simulink model "demon_sim1"  (R2021b)
settings: Solver=VariableStepAuto  StartTime=0.0  StopTime=1.0  RelTol=1e-3
settings Model: Creator=Саня  LastModifiedBy=roman

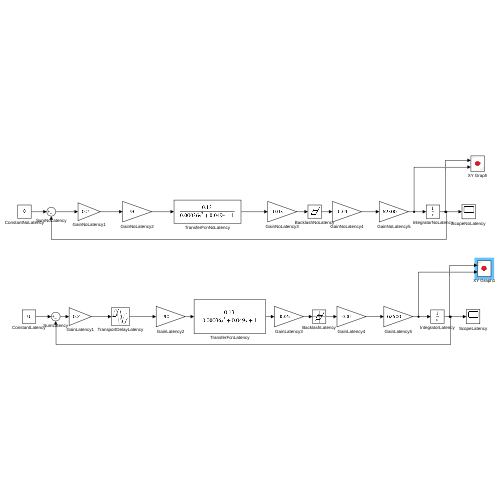
[thumbnail: Simulink's stored preview of the top-level diagram]
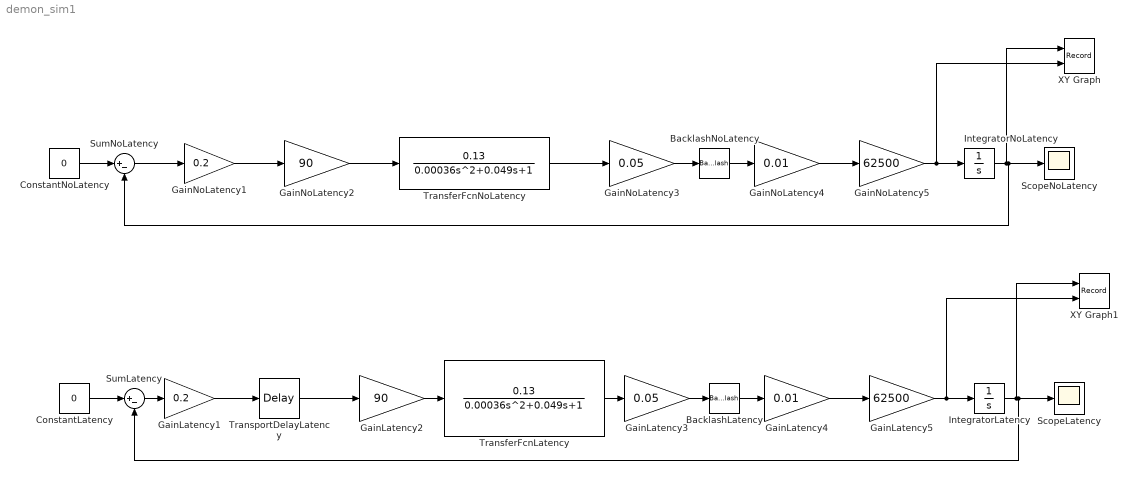
== system demon_sim1 ==
  BacklashLatency : Backlash  BacklashWidth=1e-6
  BacklashNoLatency : Backlash  BacklashWidth=1e-6
  ConstantLatency : Constant  Value=0
  ConstantNoLatency : Constant  Value=0
  GainLatency1 : Gain  Gain=0.2
  GainLatency2 : Gain  Gain=90
  GainLatency3 : Gain  Gain=0.05
  GainLatency4 : Gain  Gain=0.01
  GainLatency5 : Gain  Gain=62500
  GainNoLatency1 : Gain  Gain=0.2
  GainNoLatency2 : Gain  Gain=90  ParamDataTypeStr=double
  GainNoLatency3 : Gain  Gain=0.05
  GainNoLatency4 : Gain  Gain=0.01
  GainNoLatency5 : Gain  Gain=62500
  IntegratorLatency : Integrator  InitialCondition=13600
  IntegratorNoLatency : Integrator  InitialCondition=13600
  ScopeLatency : Scope
  ScopeNoLatency : Scope
  SumLatency : Sum  Inputs=|+-
  SumNoLatency : Sum  Inputs=|+-
  TransferFcnLatency : TransferFcn  Numerator=0.13  Denominator=[0.00036 0.049 1]
  TransferFcnNoLatency : TransferFcn  Numerator=0.13  Denominator=[0.00036 0.049 1]
  TransportDelayLatency : TransportDelay  DelayTime=0.007
  XY Graph : Record  FileSettingsInternal="{\"entries\":[{\"content\":{\"excelSettings\":{\"content\":{},\"type\":\"Streamout.ExcelSettings\"}},\"type\":\"Streamout.FileSettingStorage\",\"uuid\":\"85584950-9539-4766-aa37-add827a93c23\"}],\"packageUris\":[\"http://schema.mathworks.com/mf0/streamout_blocks/R2020a\"],\"version\":\"1.0\"}"  Layout=[1 1]  SignalsInternal="{\"entries\":[{\"content\":{\"signals\":[{\"content\":{\"blockPath\":[\"demon_sim1/XY Graph\"],\"channel\":[],\"dimensions\":[1],\"domain\":\"demon_sim1/XY Graph\",\"lineColor\":\"#a2142f\",\"plots\":[1],\"port\":1,\"sid\":[\"\"],\"signalID\":200,\"signalName\":\"IntegratorNoLatency\"},\"type\":\"RecordBlkView.Signal\",\"uuid\":\"3aafaa66-943e-4c22-807d-fb5c4517377f\"},{\"content\":{\"blockPath\":[\"demon_sim1/XY Graph\"],\"channel\":[],\"dimensions\":[1],\"domain\":\"demon_sim1/XY Graph\",\"lineColor\":\"#139fff\",\"plots\":[1],\"port\":2,\"sid\":[\"\"],\"signalID\":204,\"signalName\":\"GainNoLatency5\"},\"type\":\"RecordBlkView.Signal\",\"uuid\":\"d76adb1c-50bd-47ef-adcd-d5b8faf760cc\"}]},\"type\":\"RecordBlkView.InputSignals\",\"uuid\":\"cacb30a2-dbfc-4da8-b6af-6650a1eb4fe7\"}],\"packageUris\":[\"http://schema.mathworks.com/mf0/streamout_blocks/R2020a\"],\"version\":\"1.0\"}"  VisualizationBindings="{\"xyplotplugin\":{\"info\":[{\"series\":[{\"bindingParametersList\":[{\"parameter\":\"X-Axis\",\"signalID\":200,\"signalName\":\"IntegratorNoLatency\"},{\"parameter\":\"Y-Axis\",\"signalID\":204,\"signalName\":\"GainNoLatency5\"}],\"seriesID\":26025}],\"subplotID\":1}]}}"  CompatibilityTag=XY  st=-1
  XY Graph1 : Record  FileSettingsInternal="{\"entries\":[{\"content\":{\"excelSettings\":{\"content\":{},\"type\":\"Streamout.ExcelSettings\"}},\"type\":\"Streamout.FileSettingStorage\",\"uuid\":\"4e8ce50e-711d-469f-a9bf-3af147a9d404\"}],\"packageUris\":[\"http://schema.mathworks.com/mf0/streamout_blocks/R2020a\"],\"version\":\"1.0\"}"  Layout=[1 1]  SignalsInternal="{\"entries\":[{\"content\":{\"signals\":[{\"content\":{\"blockPath\":[\"demon_sim1/XY Graph1\"],\"channel\":[],\"dimensions\":[1],\"domain\":\"demon_sim1/XY Graph1\",\"lineColor\":\"#a2142f\",\"plots\":[1],\"port\":1,\"sid\":[\"\"],\"signalID\":192,\"signalName\":\"IntegratorLatency\"},\"type\":\"RecordBlkView.Signal\",\"uuid\":\"9a7620e4-e07a-4723-8688-f624d0f8ce6b\"},{\"content\":{\"blockPath\":[\"demon_sim1/XY Graph1\"],\"channel\":[],\"dimensions\":[1],\"domain\":\"demon_sim1/XY Graph1\",\"lineColor\":\"#139fff\",\"plots\":[1],\"port\":2,\"sid\":[\"\"],\"signalID\":196,\"signalName\":\"GainLatency5\"},\"type\":\"RecordBlkView.Signal\",\"uuid\":\"47450dd0-2938-4395-a05b-5bef7458cd1c\"}]},\"type\":\"RecordBlkView.InputSignals\",\"uuid\":\"55e4c802-81bf-4e31-93e3-04cc4471a003\"}],\"packageUris\":[\"http://schema.mathworks.com/mf0/streamout_blocks/R2020a\"],\"version\":\"1.0\"}"  VisualizationBindings="{\"xyplotplugin\":{\"info\":[{\"series\":[{\"bindingParametersList\":[{\"parameter\":\"X-Axis\",\"signalID\":192,\"signalName\":\"IntegratorLatency\"},{\"parameter\":\"Y-Axis\",\"signalID\":196,\"signalName\":\"GainLatency5\"}],\"seriesID\":1537}],\"subplotID\":1}]}}"  CompatibilityTag=XY  st=-1
  wires:
  ConstantNoLatency/1 -> SumNoLatency/1
  SumNoLatency/1 -> GainNoLatency1/1
  GainNoLatency1/1 -> GainNoLatency2/1
  GainNoLatency2/1 -> TransferFcnNoLatency/1
  TransferFcnNoLatency/1 -> GainNoLatency3/1
  GainNoLatency3/1 -> BacklashNoLatency/1
  BacklashNoLatency/1 -> GainNoLatency4/1
  GainNoLatency4/1 -> GainNoLatency5/1
  GainNoLatency5/1 -> XY Graph/2, IntegratorNoLatency/1
  IntegratorNoLatency/1 -> XY Graph/1, SumNoLatency/2, ScopeNoLatency/1
  GainLatency3/1 -> BacklashLatency/1
  TransferFcnLatency/1 -> GainLatency3/1
  GainLatency2/1 -> TransferFcnLatency/1
  BacklashLatency/1 -> GainLatency4/1
  SumLatency/1 -> GainLatency1/1
  ConstantLatency/1 -> SumLatency/1
  IntegratorLatency/1 -> XY Graph1/1, SumLatency/2, ScopeLatency/1
  GainLatency5/1 -> XY Graph1/2, IntegratorLatency/1
  GainLatency4/1 -> GainLatency5/1
  TransportDelayLatency/1 -> GainLatency2/1
  GainLatency1/1 -> TransportDelayLatency/1
